simulink model "signal_characterization_test"  (R2026a)
settings: Solver=VariableStepAuto  StopTime=10  MaxStep=0.001
settings Model: Creator=USUARIO  LastModifiedBy=osganig

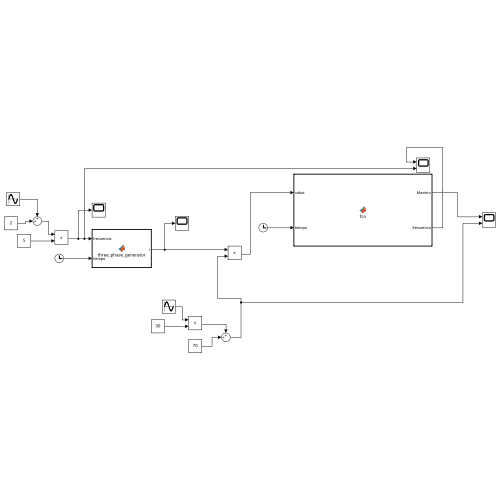
[thumbnail: Simulink's stored preview of the top-level diagram]
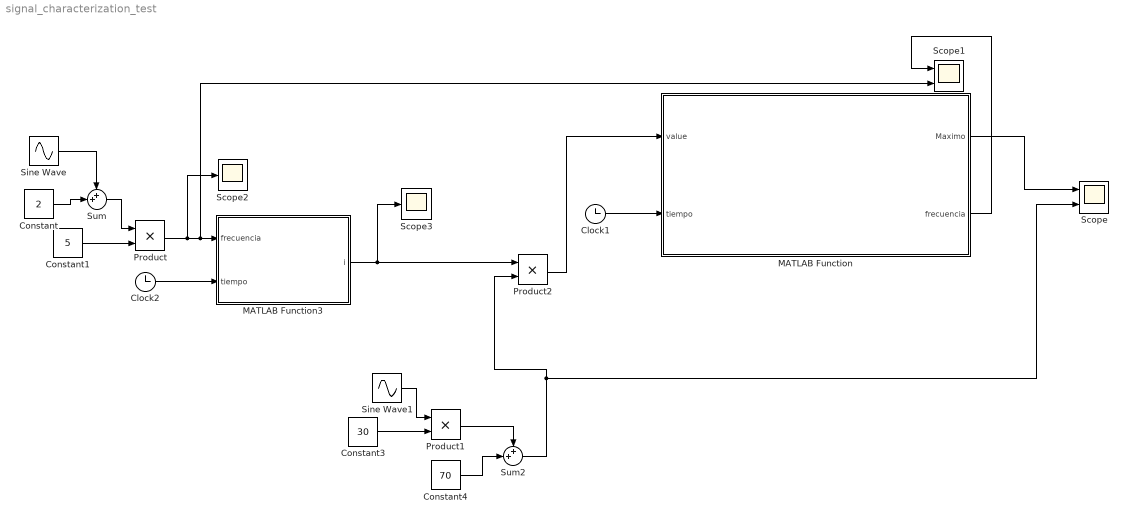
== system signal_characterization_test ==
  Clock1 : Clock
  Clock2 : Clock
  Constant : Constant  Value=2
  Constant1 : Constant  Value=5
  Constant3 : Constant  Value=30
  Constant4 : Constant  Value=70
  MATLAB Function : MATLAB Function  TreatAsAtomicUnit=on
  MATLAB Function3 : MATLAB Function  TreatAsAtomicUnit=on
  Product : Product
  Product1 : Product
  Product2 : Product
  Scope : Scope  NumInputPorts=2
      settings: ActiveDisplayYMinimum=-49.747021041982194  ActiveDisplayYMaximum=174.462580641694
  Scope1 : Scope  NumInputPorts=2
      settings: ActiveDisplayYMinimum=-9.525723529201489  ActiveDisplayYMaximum=22.514721970798572
  Scope2 : Scope
      settings: ActiveDisplayYMinimum=-1  ActiveDisplayYMaximum=1  DataLoggingVariableName=ScopeData2
  Scope3 : Scope
      settings: ActiveDisplayYMinimum=0.5686330217131228  ActiveDisplayYMaximum=0.92021016505543374  DataLoggingVariableName=ScopeData3
  Sine Wave : Sin  SampleTime=0
  Sine Wave1 : Sin  Frequency=2  SampleTime=0
  Sum : Sum  Inputs=++|
  Sum2 : Sum  Inputs=++|
  wires:
  MATLAB Function/1(Maximo) -> Scope/1
  MATLAB Function3/1(i) -> Scope3/1, Product2/1
  Clock1/1 -> MATLAB Function/2(tiempo)
  Clock2/1 -> MATLAB Function3/2(tiempo)
  Sine Wave/1 -> Sum/1
  Constant/1 -> Sum/2
  Product/1 -> Scope1/2, MATLAB Function3/1(frecuencia), Scope2/1
  Sum/1 -> Product/1
  Constant1/1 -> Product/2
  Constant3/1 -> Product1/2
  Sine Wave1/1 -> Product1/1
  Constant4/1 -> Sum2/2
  Product1/1 -> Sum2/1
  Sum2/1 -> Scope/2, Product2/2
  Product2/1 -> MATLAB Function/1(value)
  MATLAB Function/2(frecuencia) -> Scope1/1

== matlab function signal_characterization_test/MATLAB Function3 ==
  settings: updateMethod=DISCRETE
  data: i output; frecuencia input; tiempo input
function i = three_phase_generator(frecuencia, tiempo)
persistent fase
    if isempty(fase)
        fase=0;
    end
persistent t_1
    if isempty(t_1)
        t_1=0;
    end
periodo = 1/frecuencia;
dt = tiempo-t_1;
dfase = dt/periodo*2*pi;
fase = fase + dfase;
if fase>=2*pi
    fase=0;
end
u = sin(fase);
v = sin(fase + 2*pi/3);
w = sin(fase + 4*pi/3);
i = [u, v, w];
t_1=tiempo;

== matlab function signal_characterization_test/MATLAB Function ==
  data: value input; Maximo output; tiempo input; frecuencia output
function [Maximo,frecuencia]= fcn(value, tiempo)
 % Calculate Frequency and max peak

    frecuencia = frecuency_calculator(value, tiempo);
    Maximo = maximum_calculator(frecuencia, value, tiempo);

end

% Calculate Frequency
function frecuencia = frecuency_calculator(value, tiempo)
    persistent signo
    if isempty(signo)
       signo = [0 0 0]; 
    end
    persistent t_inicio
    if isempty(t_inicio)
       t_inicio = [0 0 0];
    end
    persistent frecuencia_acc
    if isempty(frecuencia_acc)
       frecuencia_acc = 1;
    end
    
    frecuencia = frecuencia_acc;
    for i = 1:3
        if signo(i) == 0
            if value(i) >= 0 
                signo(i) = 1;
            else
                signo(i) = 2;
            end
            t_inicio(i) = tiempo;
        end
        
        if signo(i) == 1
            if value(i) <= 0
                frecuencia = 1 / (2 * (tiempo - t_inicio(i)));
                frecuencia_acc = frecuencia;
                signo(i) = 0;
            end
        end
        
        if signo(i) == 2
            if value(i) >= 0
                frecuencia = 1 / (2 * (tiempo - t_inicio(i)));
                frecuencia_acc = frecuencia;
                signo(i) = 0;
            end
        end
    end
end
% Calculate Max value
function Maximo = maximum_calculator(frecuencia, valor, tiempo)
    persistent antiguo_maximo
    if isempty(antiguo_maximo)
       antiguo_maximo = 0;
    end
    persistent t_maximo
    if isempty(t_maximo)
       t_maximo = 0;
    end
    
    maximo = [0 0 0];
    periodo = 1 / abs(frecuencia) / 3;
    for i = 1:3
        if abs(valor(i)) >= antiguo_maximo
            maximo(i) = abs(valor(i));
            antiguo_maximo = abs(valor(i));
            t_maximo = tiempo;
        else
            maximo(i) = antiguo_maximo;
            if tiempo > t_maximo + periodo
                maximo(i) = abs(valor(i));
                antiguo_maximo = abs(valor(i));
                t_maximo = tiempo;
            end
        end
    end
    Maximo = max(maximo);
end
